simulink model "VehicleDynamics"  (Simulink 8.7)
settings: Solver=ode45  StartTime=0.0  StopTime=10.0  RelTol=1e-3
values from neighbouring files (symbols this model uses):
  Av = 2.75    [InitiateModel.m]
  Cd = 0.29    [InitiateModel.m]
  Cr = 0.01    [InitiateModel.m]
  Fe_max = Pe_max/Vbase    (= 5965.16344548)    [InitiateModel.m]
  Mv = 1620    [InitiateModel.m]
  Pe_max = Pe_max*eff    (= 80000)    [InitiateModel.m]
  rho_air = 1.204    [InitiateModel.m]
settings Model: Creator=Dragan  LastModifiedBy=Dragan
settings DataIOCC: SignalLoggingSaveFormat=ModelDataLogs
settings OptimizationCC: ExpressionDepthLimit=2147483647
settings DebuggingCC: SolverPrmCheckMsg=warning  FcnCallInpInsideContextMsg=EnableAllAsWarning  StateNameClashWarn=warning

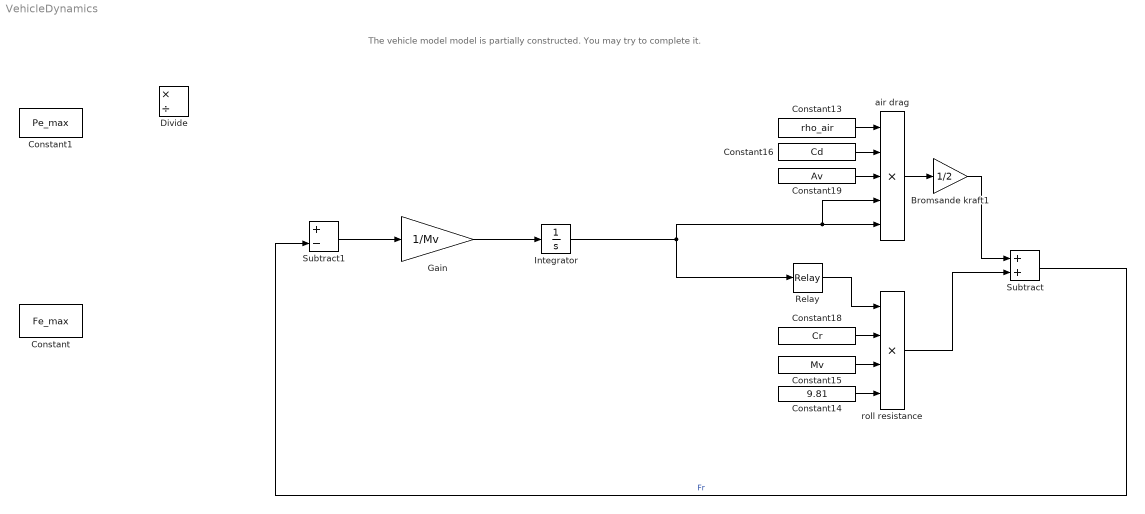
== system VehicleDynamics ==
  note: The vehicle model model is partially constructed. You may try to complete it.
  Bromsande kraft1 : Gain  Gain=1/2  SaturateOnIntegerOverflow=on  OutDataTypeStr=Inherit: Same as input  ParamDataTypeStr=Inherit: Same as input
  Constant : Constant  Value=Fe_max
  Constant1 : Constant  Value=Pe_max
  Constant13 : Constant  Value=rho_air
  Constant14 : Constant  Value=9.81
  Constant15 : Constant  Value=Mv
  Constant16 : Constant  Value=Cd
  Constant18 : Constant  Value=Cr
  Constant19 : Constant  Value=Av
  Divide : Product  Inputs=*/
  Gain : Gain  Gain=1/Mv
  Integrator : Integrator
  Relay : Relay
  Subtract : Sum
  Subtract1 : Sum  Inputs=+-
  air drag : Product  Inputs=5  SaturateOnIntegerOverflow=on  InputSameDT=on  OutDataTypeStr=Inherit: Same as first input
  roll resistance : Product  Inputs=4  SaturateOnIntegerOverflow=on  InputSameDT=on  OutDataTypeStr=Inherit: Same as first input
  wires:
  Constant19/1 -> air drag/3
  Constant16/1 -> air drag/2
  Constant13/1 -> air drag/1
  air drag/1 -> Bromsande kraft1/1
  Relay/1 -> roll resistance/1
  Constant14/1 -> roll resistance/4
  Constant15/1 -> roll resistance/3
  Constant18/1 -> roll resistance/2
  Bromsande kraft1/1 -> Subtract/1
  roll resistance/1 -> Subtract/2
  Subtract/1 -> Subtract1/2  "Fr"
  Subtract1/1 -> Gain/1
  Gain/1 -> Integrator/1
  Integrator/1 -> Relay/1, air drag/5, air drag/4
